simulink model "drymodel"  (Simulink 7.6)
settings: Solver=ode45  StartTime=0.0  StopTime=inf  RelTol=1e-3
values from neighbouring files (symbols this model uses):
  s = evalin('base','s')    [GUI_MT218.m]
undefined symbols (not defined in the file or in its folder): TS_boat
libraries: simulink x5
settings Model: Creator=Andries  LastModifiedBy=Andries

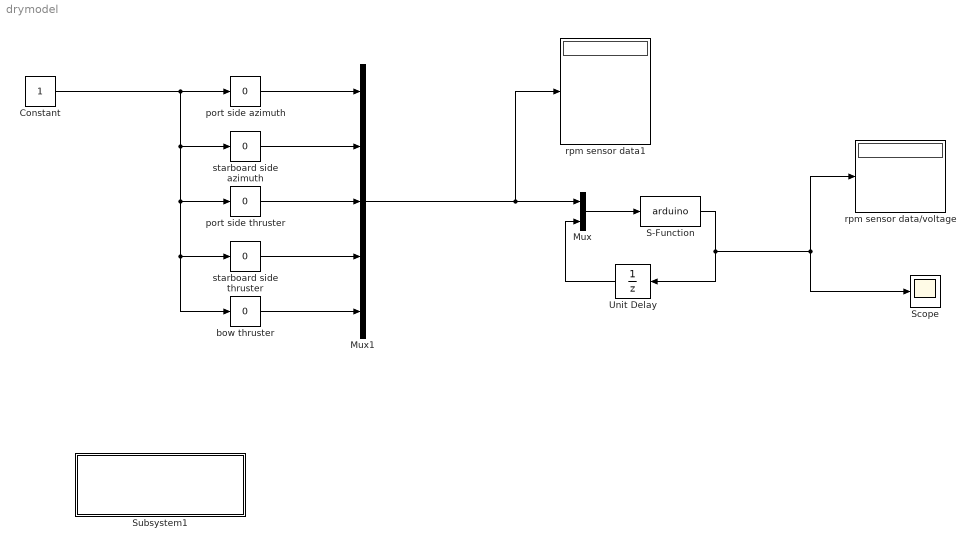
== system drymodel ==
  Constant : Constant
  Mux : Mux  Inputs=2
  Mux1 : Mux  Inputs=5
  S-Function : S-Function  FunctionName=arduino  Parameters=TS_boat,s  EnableBusSupport=off
  Scope : Scope
      settings: YMin=0  YMax=16
  Subsystem1 : Subsystem
      mask Display:
      | if evalin('base','exist(''boat'')');
      |     set_param(gcb,'BackgroundColor','Green')
      |     disp(['connected to: ',evalin('base','boat.name')]);
      | else
      |     disp('no boat connected')
      |     set_param(gcb,'BackgroundColor','Red')
      |     color('red')
      | end
  Unit Delay : UnitDelay  SampleTime=-1
  bow thruster : simulink/Math Operations/Slider Gain  SystemSampleTime=-1  low=-1  gain=0  high=1
  port side azimuth : simulink/Math Operations/Slider Gain  SystemSampleTime=-1  low=-1  gain=0  high=1
  port side thruster : simulink/Math Operations/Slider Gain  SystemSampleTime=-1  low=-1  gain=0  high=1
  rpm sensor data/voltage : Display
  rpm sensor data1 : Display
  starboard side azimuth : simulink/Math Operations/Slider Gain  SystemSampleTime=-1  low=-1  gain=0  high=1
  starboard side thruster : simulink/Math Operations/Slider Gain  SystemSampleTime=-1  low=-1  gain=0  high=1
  wires:
  Constant/1 -> port side azimuth/1, starboard side azimuth/1, port side thruster/1, starboard side thruster/1, bow thruster/1
  port side azimuth/1 -> Mux1/1
  starboard side azimuth/1 -> Mux1/2
  port side thruster/1 -> Mux1/3
  starboard side thruster/1 -> Mux1/4
  bow thruster/1 -> Mux1/5
  Mux1/1 -> Mux/1, rpm sensor data1/1
  Mux/1 -> S-Function/1
  Unit Delay/1 -> Mux/2
  S-Function/1 -> Unit Delay/1, rpm sensor data/voltage/1, Scope/1

== system drymodel/Subsystem1 ==
